simulink model "PenduloInvertidoLINEAL"  (R2018a)
settings: Solver=ode4  StartTime=0.0  StopTime=10.0  FixedStep=0.01  RelTol=1e-3
values from neighbouring files (symbols this model uses):
  g = 9.81    [ParametrosPenduloInvertido.m]
  l = 0.45    [ParametrosPenduloInvertido.m]
  M = 2    [ParametrosPenduloInvertido.m]
  m = 0.5    [ParametrosPenduloInvertido.m]
settings Model: Creator=Benjamin Nicolas  LastModifiedBy=Benjamin Nicolas

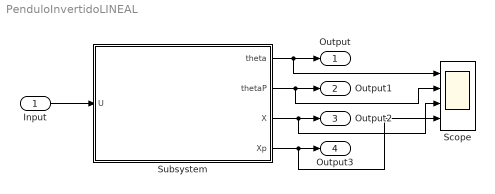
== system PenduloInvertidoLINEAL ==
  Input : Inport
  Scope : Scope  NumInputPorts=4
  Subsystem : Subsystem
  Output : Outport
  Output1 : Outport  Port=2
  Output2 : Outport  Port=3
  Output3 : Outport  Port=4
  wires:
  Input/1 -> Subsystem/1(U)
  Subsystem/1(theta) -> Scope/1, Output/1
  Subsystem/2(thetaP) -> Scope/2, Output1/1
  Subsystem/3(X) -> Scope/3, Output2/1
  Subsystem/4(Xp) -> Scope/4, Output3/1

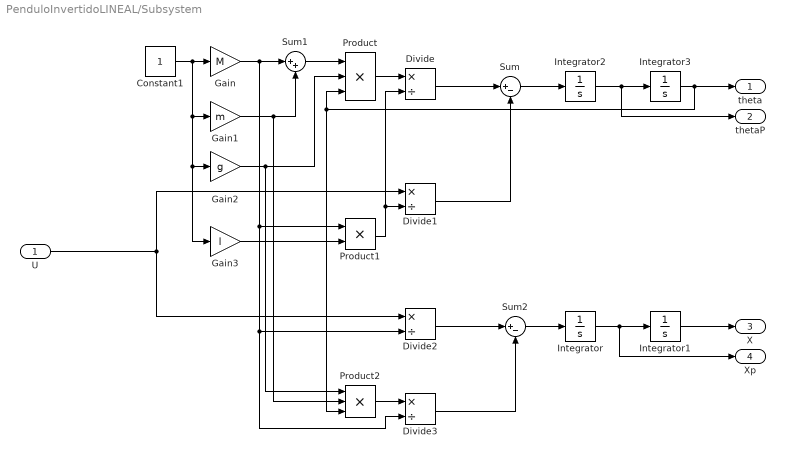
== system PenduloInvertidoLINEAL/Subsystem ==
  U : Inport
  Constant1 : Constant
  Divide{,1..3} (4 alike) : Product  Inputs=*/
  Gain : Gain  Gain=M
  Gain1 : Gain  Gain=m
  Gain2 : Gain  Gain=g
  Gain3 : Gain  Gain=l
  Integrator{,1..3} (4 alike) : Integrator  InitialCondition=pi/8
  Product : Product  Inputs=3
  Product1 : Product
  Product2 : Product  Inputs=3
  Sum : Sum  Inputs=|+-
  Sum1 : Sum  Inputs=|++
  Sum2 : Sum  Inputs=|+-
  theta : Outport
  thetaP : Outport  Port=2
  X : Outport  Port=3
  Xp : Outport  Port=4
  wires:
  Divide1/1 -> Sum/2
  Gain/1 -> Divide3/2, Divide2/2, Product1/1, Sum1/1
  Divide/1 -> Sum/1
  Gain1/1 -> Product2/2, Sum1/2
  U/1 -> Divide1/1, Divide2/1
  Constant1/1 -> Gain3/1, Gain2/1, Gain1/1, Gain/1
  Integrator/1 -> Xp/1, Integrator1/1
  Divide3/1 -> Sum2/2
  Integrator2/1 -> thetaP/1, Integrator3/1
  Gain2/1 -> Product2/1, Product/2
  Integrator3/1 -> theta/1, Product2/3, Product/3
  Sum2/1 -> Integrator/1
  Product1/1 -> Divide/2, Divide1/2
  Product2/1 -> Divide3/1
  Integrator1/1 -> X/1
  Product/1 -> Divide/1
  Sum1/1 -> Product/1
  Divide2/1 -> Sum2/1
  Sum/1 -> Integrator2/1
  Gain3/1 -> Product1/2
